simulink model "pract_3"  (R2020b)
settings: Solver=VariableStepAuto  StartTime=0.0  StopTime=10.0  RelTol=1e-3
libraries: powerlib_meascontrol x4
settings Model: Creator=Egor  LastModifiedBy=Egor

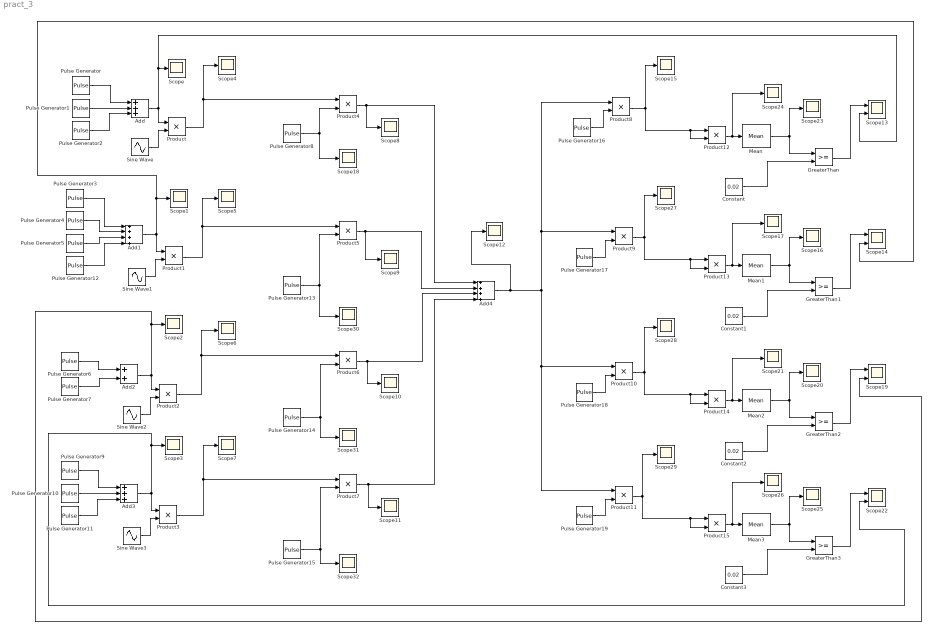
== system pract_3 ==
  Add : Sum  Inputs=+++
  Add1 : Sum  Inputs=++++
  Add2 : Sum
  Add3 : Sum  Inputs=+++
  Add4 : Sum  Inputs=++++
  Constant{,1..3} (4 alike) : Constant  Value=0.02
  GreaterThan{,1..3} (4 alike) : RelationalOperator  OutDataTypeStr=boolean  RndMeth=Simplest
  Mean{,1..3} (4 alike) : powerlib_meascontrol/Measurements/Mean  Freq=100  Vinit=0  Ts=0
  Product{,1..15} (16 alike) : Product
  Pulse Generator : DiscretePulseGenerator  PulseType=Time based  Period=1  PulseWidth=10
  Pulse Generator1 : DiscretePulseGenerator  PulseType=Time based  Period=1  PulseWidth=10  PhaseDelay=0.4
  Pulse Generator10 : DiscretePulseGenerator  PulseType=Time based  Period=1  PulseWidth=10  PhaseDelay=0.2
  Pulse Generator11 : DiscretePulseGenerator  PulseType=Time based  Period=1  PulseWidth=10  PhaseDelay=0.3
  Pulse Generator12 : DiscretePulseGenerator  PulseType=Time based  Period=1  PulseWidth=10  PhaseDelay=0.5
  Pulse Generator13 : DiscretePulseGenerator  PulseType=Time based  Period=0.01  PulseWidth=25  PhaseDelay=0.0025
  Pulse Generator14 : DiscretePulseGenerator  PulseType=Time based  Period=0.01  PulseWidth=25  PhaseDelay=0.005
  Pulse Generator15 : DiscretePulseGenerator  PulseType=Time based  Period=0.01  PulseWidth=25  PhaseDelay=0.0075
  Pulse Generator16 : DiscretePulseGenerator  PulseType=Time based  Period=0.01  PulseWidth=25
  Pulse Generator17 : DiscretePulseGenerator  PulseType=Time based  Period=0.01  PulseWidth=25  PhaseDelay=0.0025
  Pulse Generator18 : DiscretePulseGenerator  PulseType=Time based  Period=0.01  PulseWidth=25  PhaseDelay=0.005
  Pulse Generator19 : DiscretePulseGenerator  PulseType=Time based  Period=0.01  PulseWidth=25  PhaseDelay=0.0075
  Pulse Generator2 : DiscretePulseGenerator  PulseType=Time based  Period=1  PulseWidth=10  PhaseDelay=0.5
  Pulse Generator3 : DiscretePulseGenerator  PulseType=Time based  Period=1  PulseWidth=10
  Pulse Generator4 : DiscretePulseGenerator  PulseType=Time based  Period=1  PulseWidth=10  PhaseDelay=0.2
  Pulse Generator5 : DiscretePulseGenerator  PulseType=Time based  Period=1  PulseWidth=10  PhaseDelay=0.4
  Pulse Generator6 : DiscretePulseGenerator  PulseType=Time based  Period=1  PulseWidth=10  PhaseDelay=0.1
  Pulse Generator7 : DiscretePulseGenerator  PulseType=Time based  Period=1  PulseWidth=10  PhaseDelay=0.3
  Pulse Generator8 : DiscretePulseGenerator  PulseType=Time based  Period=0.01  PulseWidth=25
  Pulse Generator9 : DiscretePulseGenerator  PulseType=Time based  Period=1  PulseWidth=10  PhaseDelay=0.1
  Scope{,1..12,15..18,20..21,23..32} (29 alike) : Scope
  Scope{13..14,19,22} (4 alike) : Scope  NumInputPorts=2
  Sine Wave{,1..3} (4 alike) : Sin  Frequency=500  SampleTime=0.0001
  wires:
  Pulse Generator1/1 -> Add/2
  Pulse Generator2/1 -> Add/3
  Pulse Generator/1 -> Add/1
  Pulse Generator3/1 -> Add1/1
  Pulse Generator5/1 -> Add1/3
  Pulse Generator4/1 -> Add1/2
  Pulse Generator7/1 -> Add2/2
  Pulse Generator6/1 -> Add2/1
  Pulse Generator9/1 -> Add3/1
  Pulse Generator11/1 -> Add3/3
  Pulse Generator10/1 -> Add3/2
  Pulse Generator12/1 -> Add1/4
  Sine Wave/1 -> Product/2
  Product/1 -> Product4/1, Scope4/1
  Product1/1 -> Scope5/1, Product5/1
  Sine Wave1/1 -> Product1/2
  Sine Wave2/1 -> Product2/2
  Product2/1 -> Product6/1, Scope6/1
  Product3/1 -> Product7/1, Scope7/1
  Sine Wave3/1 -> Product3/2
  Pulse Generator8/1 -> Scope18/1, Product4/2
  Product4/1 -> Add4/1, Scope8/1
  Product5/1 -> Add4/2, Scope9/1
  Pulse Generator13/1 -> Scope30/1, Product5/2
  Pulse Generator14/1 -> Product6/2, Scope31/1
  Product7/1 -> Add4/4, Scope11/1
  Pulse Generator15/1 -> Scope32/1, Product7/2
  Product6/1 -> Add4/3, Scope10/1
  Add4/1 -> Scope12/1, Product9/1, Product8/1, Product11/1, Product10/1
  Pulse Generator16/1 -> Product8/2
  Pulse Generator17/1 -> Product9/2
  Pulse Generator18/1 -> Product10/2
  Pulse Generator19/1 -> Product11/2
  Product8/1 -> Product12/2, Product12/1, Scope15/1
  Product12/1 -> Mean/1, Scope24/1
  Constant/1 -> GreaterThan/2
  GreaterThan/1 -> Scope13/1
  Mean/1 -> GreaterThan/1, Scope23/1
  Mean1/1 -> Scope16/1, GreaterThan1/1
  GreaterThan1/1 -> Scope14/1
  Constant1/1 -> GreaterThan1/2
  Product13/1 -> Scope17/1, Mean1/1
  Product9/1 -> Scope27/1, Product13/1, Product13/2
  Product10/1 -> Scope28/1, Product14/2, Product14/1
  Product14/1 -> Mean2/1, Scope21/1
  Constant2/1 -> GreaterThan2/2
  GreaterThan2/1 -> Scope19/1
  Mean2/1 -> GreaterThan2/1, Scope20/1
  Mean3/1 -> Scope25/1, GreaterThan3/1
  GreaterThan3/1 -> Scope22/1
  Constant3/1 -> GreaterThan3/2
  Product15/1 -> Scope26/1, Mean3/1
  Product11/1 -> Scope29/1, Product15/1, Product15/2
  Add/1 -> Product/1, Scope13/2, Scope/1
  Add1/1 -> Product1/1, Scope1/1, Scope14/2
  Add2/1 -> Product2/1, Scope19/2, Scope2/1
  Add3/1 -> Product3/1, Scope22/2, Scope3/1
